simulink subsystem "Features_System"  (R2020b)
settings: Solver=VariableStepAuto  StartTime=0.0  StopTime=10.0  RelTol=1e-3
model mask{s0=[], noise_power=0, noise_sample_time=0.1}
  mask prompts: noise_power "Noise Power"; noise_sample_time "Noise Sample Time"
libraries: simulink x1
settings Model: Creator=marco  LastModifiedBy=marco

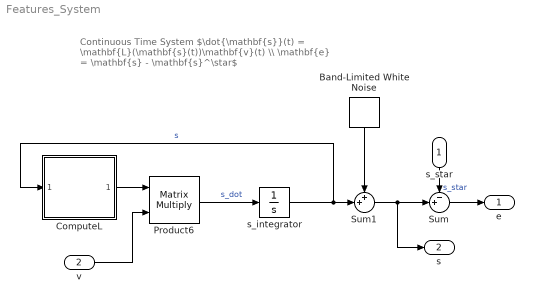
== system Features_System ==
  note: Continuous Time System
      | $\dot{\mathbf{s}}(t) = \mathbf{L}(\mathbf{s}(t))\mathbf{v}(t) \\ \mathbf{e} = \mathbf{s} - \mathbf{s}^\star$
  s_star : Inport
  v : Inport  Port=2
  Band-Limited White Noise : simulink/Sources/Band-Limited White Noise  Cov=noise_power * ones(size(s0))  Ts=noise_sample_time  seed=round(rand(size(s0))*1000)
  ComputeL : Subsystem  ReferencedSubsystem=ComputeL
  Product6 : Product  Multiplication=Matrix(*)
  Sum : Sum  Inputs=-+|
  Sum1 : Sum  Inputs=++|
  s_integrator : Integrator  InitialCondition=s0
  e : Outport
  s : Outport  Port=2
  wires:
  Band-Limited White Noise/1 -> Sum1/1
  Sum1/1 -> s/1, Sum/2
  ComputeL/1 -> Product6/1
  Sum/1 -> e/1
  v/1 -> Product6/2
  s_star/1 -> Sum/1  "s_star"
  s_integrator/1 -> Sum1/2, ComputeL/1  "s"
  Product6/1 -> s_integrator/1  "s_dot"
